simulink model "rtwdemo_dowhilesf"  (Simulink 7.1)
settings: Solver=FixedStepDiscrete  StartTime=0.0  StopTime=10  FixedStep=.01  RelTol=1e-3
settings Model: Creator=ajayaram  LastModifiedBy=ajayaram
settings OptimizationCC: InlineParams=on  OptimizeModelRefInitCode=on  LifeSpan=1
settings DebuggingCC: SaveWithParameterizedLinksMsg=none
settings RTWCC: SystemTargetFile=ert.tlc  GenCodeOnly=on  GenerateMakefile=off  TemplateMakefile=ert_default_tmf  Description=Real-Time Workshop Embedded Coder (no auto configuration)  GenerateReport=on  ProcessScript=ert_make_rtw_hook  IncludeHyperlinkInReport=on  LaunchReport=on
settings CodeAppCC: GenerateComments=off  IgnoreCustomStorageClasses=off  SimulinkBlockComments=off
settings ERTTargetCC: TargetFcnLib=ansi_tfl_tmw.mat  GenerateSampleERTMain=on  InlinedParameterPlacement=NonHierarchical  ERTCustomFileTemplate=example_file_process.tlc

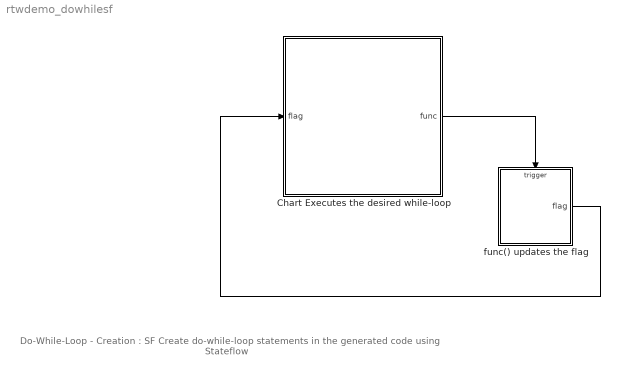
== system rtwdemo_dowhilesf ==
  note: Do-While-Loop - Creation : SF
      | Create do-while-loop statements in the
      | generated code using Stateflow
  Chart Executes the desired while-loop : Stateflow chart
      settings: RTWSystemCode=Inline
  func() updates the flag : Subsystem  RTWFcnName=func  RTWFileName=func
      settings: RTWSystemCode=Function  RTWFcnNameOpts=User specified  RTWFileNameOpts=User specified
  wires:
  Chart Executes the desired while-loop/1(func) -> func() updates the flag/Trigger
  func() updates the flag/1(flag) -> Chart Executes the desired while-loop/1(flag)

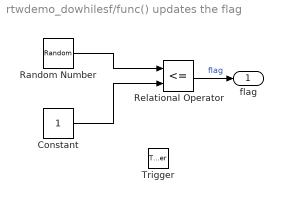
== system rtwdemo_dowhilesf/func() updates the flag ==
  Trigger : TriggerPort  TriggerType=function-call
  Constant : Constant  OutDataType=sfix(16)  OutScaling=2^0
  Random Number : RandomNumber
  Relational Operator : RelationalOperator  Operator=<=  LogicOutDataTypeMode=boolean  OutDataTypeStr=boolean
  flag : Outport  OutDataType=sfix(16)  OutScaling=2^0
  wires:
  Random Number/1 -> Relational Operator/1
  Constant/1 -> Relational Operator/2
  Relational Operator/1 -> flag/1  "flag"

== stateflow chart Chart Executes the desired while-loop ==
  (junction 5) -> (junction 3) [order 2]
  (junction 4) -> (junction 5) : {
      |  func;
      |  num_iter++;
      | }
  (junction 6) -> (junction 4)
  (junction 5) -> (junction 6) [order 1] : [flag && (num_iter<=100)]
  (default) -> (junction 4) : {
      | num_iter=1;
      | }
  data: flag input boolean; num_iter local int32
  events: func output FUNCTION_CALL_EVENT
